simulink model "Moore"  (R2020b)
settings: Solver=FixedStepDiscrete  StartTime=0.0  StopTime=150  RelTol=1e-3
undefined symbols (not defined in the file): DiscIntNeverNeededParam
libraries: simulink x1
settings Model: Creator=priyaD  LastModifiedBy=priyaD

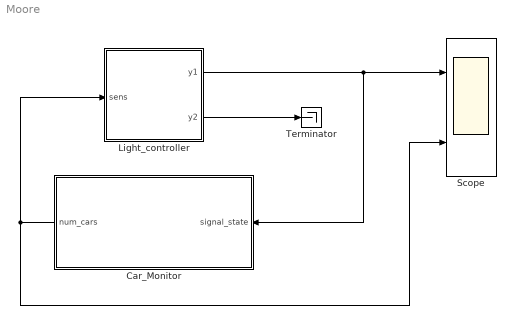
== system Moore ==
  Car_Monitor : Subsystem
  Light_controller : Stateflow chart  TreatAsAtomicUnit=on
  Scope : Scope  NumInputPorts=2
  Terminator : Terminator
  wires:
  Car_Monitor/1(num_cars) -> Light_controller/1(sens), Scope/2
  Light_controller/1(y1) -> Scope/1, Car_Monitor/1(signal_state)
  Light_controller/2(y2) -> Terminator/1

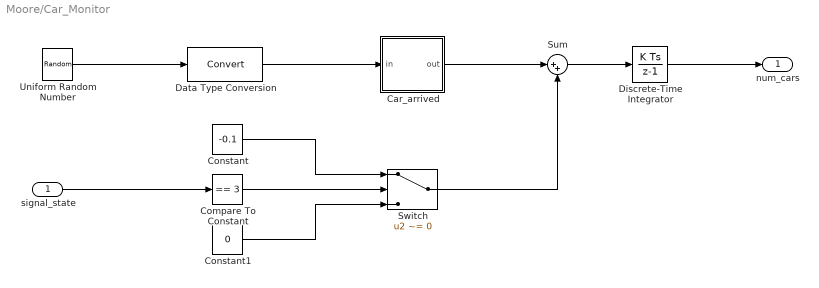
== system Moore/Car_Monitor ==
  signal_state : Inport
  Car_arrived : Stateflow chart  TreatAsAtomicUnit=on
  Compare To Constant : simulink/Logic and Bit Operations/Compare To Constant  relop===  const=3  OutDataTypeStr=boolean  ZeroCross=off
  Constant : Constant  Value=-0.1
  Constant1 : Constant  Value=0
  Data Type Conversion : DataTypeConversion
  Discrete-Time Integrator : DiscreteIntegrator  SampleTime=-1  LimitOutput=on  ICPrevOutput=DiscIntNeverNeededParam  ICPrevScaledInput=DiscIntNeverNeededParam
  Sum : Sum  Inputs=|++
  Switch : Switch  Criteria=u2 ~= 0
  Uniform Random Number : UniformRandomNumber  Minimum=0  Maximum=100  Seed=177836  SampleTime=0
  num_cars : Outport
  wires:
  signal_state/1 -> Compare To Constant/1
  Uniform Random Number/1 -> Data Type Conversion/1
  Data Type Conversion/1 -> Car_arrived/1(in)
  Compare To Constant/1 -> Switch/2
  Constant/1 -> Switch/1
  Discrete-Time Integrator/1 -> num_cars/1
  Switch/1 -> Sum/2
  Constant1/1 -> Switch/3
  Car_arrived/1(out) -> Sum/1
  Sum/1 -> Discrete-Time Integrator/1

== stateflow chart Moore/Car_Monitor/Car_arrived ==
  (default) -> (junction 1) : {out=in>98;}
  data: in input; out output

== stateflow chart Moore/Light_controller ==
  settings: stateMachineType=MOORE_MACHINE  initializeOutput=1
  state Stop
    y1 = RED;
    y2 = GREEN;
  state StopForTraffic
    y1 = RED;
    y2 = GREEN;
  state StopToGo
    y1 = RED;
    y2 = YELLOW;
  state GoToStop
    y1 = YELLOW;
    y2 = RED;
  state Go
    y1 = GREEN;
    y2 = RED;
  (default) -> Stop
  Stop -> StopForTraffic : after(20,tick)
  StopForTraffic -> StopToGo : [sens]
  StopToGo -> Go : after(3,tick)
  GoToStop -> Stop : after(3,tick)
  Go -> GoToStop : after(10,tick)
  data: GREEN constant double =3; RED constant double =1; YELLOW constant double =2; y1 output; y2 output; sens input
